simulink model "EvenOdd"  (R2016b)
settings: Solver=FixedStepDiscrete  StartTime=0.0  StopTime=30  RelTol=1e-3
libraries: simulink x1
settings Model: Creator=3essawy  LastModifiedBy=3essawy
settings OptimizationCC: DefaultParameterBehavior=Inlined
settings DebuggingCC: ParameterTunabilityLossMsg=error
settings RTWCC: SystemTargetFile=ert.tlc  GenCodeOnly=on  TemplateMakefile=ert_default_tmf  Description=Embedded Coder  GenerateReport=on  IncludeHyperlinkInReport=on  LaunchReport=on  GenerateTraceInfo=on  GenerateTraceReport=on  GenerateTraceReportSl=on  GenerateTraceReportSf=on  GenerateTraceReportEml=on
settings CodeAppCC: ForceParamTrailComments=on  IgnoreCustomStorageClasses=off  OperatorAnnotations=on  SimulinkDataObjDesc=on  SFDataObjDesc=on  MATLABFcnDesc=on  InsertBlockDesc=on  MATLABSourceComments=on
settings ERTTargetCC: TargetLangStandard=C99 (ISO)  GenerateSampleERTMain=on  InlinedParameterPlacement=NonHierarchical  ERTCustomFileTemplate=example_file_process.tlc  EnableUserReplacementTypes=on

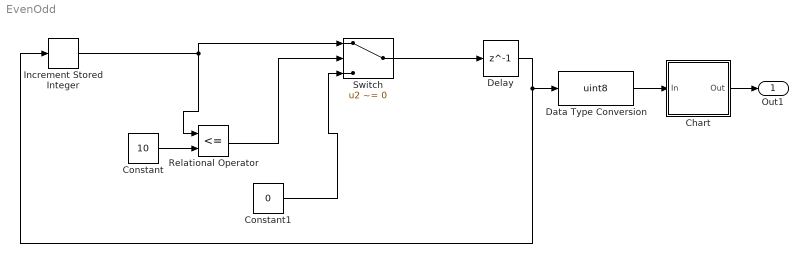
== system EvenOdd ==
  Chart : Stateflow chart  TreatAsAtomicUnit=on
  Constant : Constant  Value=10
  Constant1 : Constant  Value=0
  Data Type Conversion : DataTypeConversion  OutDataTypeStr=uint8
  Delay : Delay  DelayLength=1
  Increment Stored Integer : simulink/Additional Math & Discrete/Additional Math: Increment - Decrement/Increment Stored Integer
  Relational Operator : RelationalOperator  Operator=<=  OutDataTypeStr=boolean  RndMeth=Simplest
  Switch : Switch  Criteria=u2 ~= 0
  Out1 : Outport
  wires:
  Increment Stored Integer/1 -> Switch/1, Relational Operator/1
  Delay/1 -> Data Type Conversion/1, Increment Stored Integer/1
  Constant/1 -> Relational Operator/2
  Relational Operator/1 -> Switch/2
  Constant1/1 -> Switch/3
  Switch/1 -> Delay/1
  Chart/1(Out) -> Out1/1
  Data Type Conversion/1 -> Chart/1(In)

== stateflow chart EvenOdd/Chart ==
  state EvenOdd [function]
    (default) -> (junction 10)
    (junction 10) -> (junction 11) [order 1] : [In&0x01==1]
    (junction 10) -> (junction 12) [order 2] : {Out=2;}
    (junction 11) -> (junction 13) : {Out=1;}
    (junction 13) -> (junction 12)
    (junction 12) -> (junction 14)
  (default) -> (junction 16) : {EvenOdd();}
  data: In input; Out output double
